simulink library "SCGAnalysis_SignalGenerationLib"  (R2020b)
settings: Solver=VariableStepAuto  StartTime=0.0  StopTime=10.0  RelTol=1e-3
undefined symbols (not defined in the file or in its folder): analyses, fs
settings Model: Creator=Rafael  LastModifiedBy=Rafael

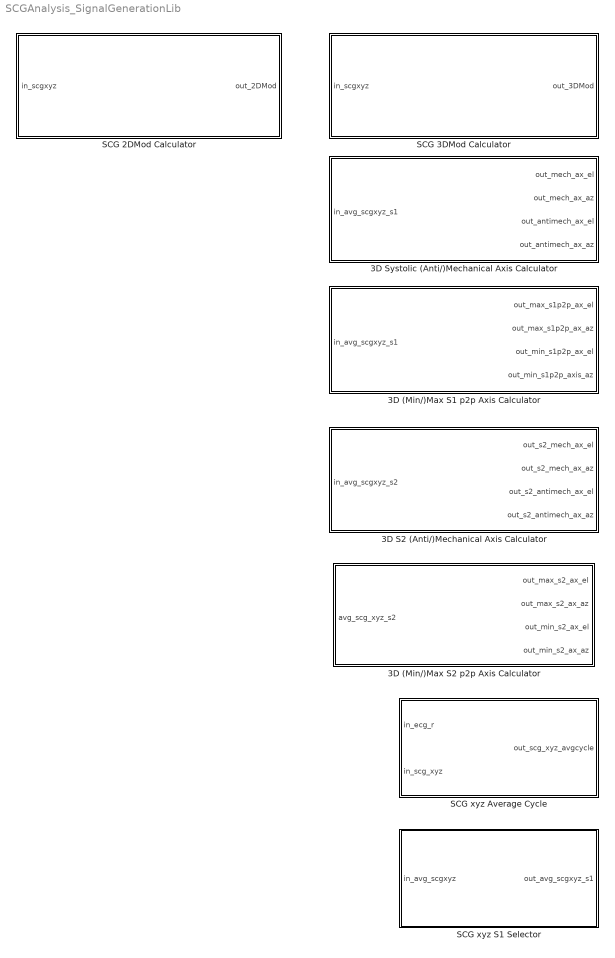
== system SCGAnalysis_SignalGenerationLib ==
  3D (Min/)Max S1 p2p Axis Calculator : Subsystem
      mask Display: image('$imagefile'); % Use "Edit Image" on toolstrip to change.
  3D (Min/)Max S2 p2p Axis Calculator : Subsystem
      mask Display: image('3D Max S2P2P Axis.png'); % Use "Edit Image" on toolstrip to change.
  3D S2 (Anti/)Mechanical Axis Calculator : Subsystem
      mask Display: image('$imagefile'); % Use "Edit Image" on toolstrip to change.
  3D Systolic (Anti/)Mechanical Axis Calculator : Subsystem
      mask Display: image('$imagefile'); % Use "Edit Image" on toolstrip to change.
  SCG 2DMod Calculator : Subsystem  mask{xyz2Dcombo=xz (transverse plane)}
      mask prompts: xyz2Dcombo "2D component combination:"
      mask init:
      | if xyz2Dcombo == 1
      |     param_2Dxyzcombo = 'xy';
      | elseif xyz2Dcombo == 2
      |     param_2Dxyzcombo = 'yz';
      | elseif xyz2Dcombo == 3
      |     param_2Dxyzcombo = 'xz';
      | end
      | 
      | assignin('base','param_2Dxyzcombo', param_2Dxyzcombo)
      mask TypeOptions xyz2Dcombo: xy (coronal plane) | yz (sagittal plane) | xz (transverse plane)
      mask DialogControl DescGroupVar Prompt: 2D Modulus Calculator
      mask DialogControl DescTextVar Prompt: Subsystem to calculate a 2D modulus signal from a user-specified combination of any two of the SCG x, y, or z components.
      mask Display: image('$imagefile'); % Use "Edit Image" on toolstrip to change.
  SCG 3DMod Calculator : Subsystem
      mask Display: image('$imagefile'); % Use "Edit Image" on toolstrip to change.
  SCG xyz Average Cycle : Subsystem
      mask Display: image('$imagefile'); % Use "Edit Image" on toolstrip to change.
  SCG xyz S1 Selector : Subsystem
      mask Display: image('Average S1.png'); % Use "Edit Image" on toolstrip to change.

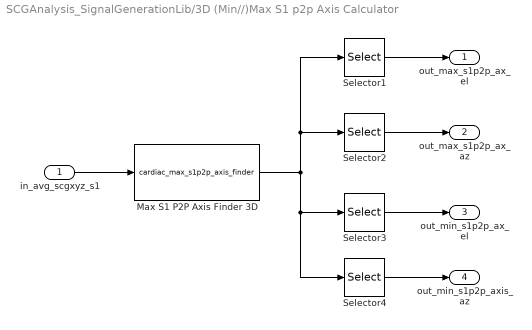
== system SCGAnalysis_SignalGenerationLib/3D (Min//)Max S1 p2p Axis Calculator ==
  in_avg_scgxyz_s1 : Inport
  Max S1 P2P Axis Finder 3D : MATLABFcn  MATLABFcn=cardiac_max_s1p2p_axis_finder  OutputDimensions=4  Output1D=off
  Selector1 : Selector  InputPortWidth=4  IndexOptions=Index vector (dialog)  Indices=[1]  OutputSizes=1
  Selector2 : Selector  InputPortWidth=4  IndexOptions=Index vector (dialog)  Indices=[2]  OutputSizes=1
  Selector3 : Selector  InputPortWidth=4  IndexOptions=Index vector (dialog)  Indices=[3]  OutputSizes=1
  Selector4 : Selector  InputPortWidth=4  IndexOptions=Index vector (dialog)  Indices=[4]  OutputSizes=1
  out_max_s1p2p_ax_el : Outport
  out_max_s1p2p_ax_az : Outport  Port=2
  out_min_s1p2p_ax_el : Outport  Port=3
  out_min_s1p2p_axis_az : Outport  Port=4
  wires:
  in_avg_scgxyz_s1/1 -> Max S1 P2P Axis Finder 3D/1
  Max S1 P2P Axis Finder 3D/1 -> Selector4/1, Selector3/1, Selector1/1, Selector2/1
  Selector1/1 -> out_max_s1p2p_ax_el/1
  Selector2/1 -> out_max_s1p2p_ax_az/1
  Selector4/1 -> out_min_s1p2p_axis_az/1
  Selector3/1 -> out_min_s1p2p_ax_el/1

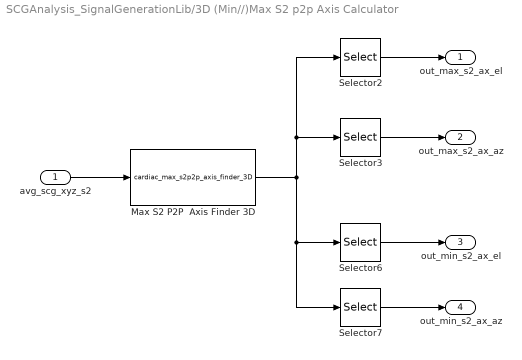
== system SCGAnalysis_SignalGenerationLib/3D (Min//)Max S2 p2p Axis Calculator ==
  avg_scg_xyz_s2 : Inport
  Max S2 P2P  Axis Finder 3D : MATLABFcn  MATLABFcn=cardiac_max_s2p2p_axis_finder_3D  OutputDimensions=4  Output1D=off
  Selector2 : Selector  InputPortWidth=4  IndexOptions=Index vector (dialog)  Indices=[1]  OutputSizes=1
  Selector3 : Selector  InputPortWidth=4  IndexOptions=Index vector (dialog)  Indices=[2]  OutputSizes=1
  Selector6 : Selector  InputPortWidth=4  IndexOptions=Index vector (dialog)  Indices=[3]  OutputSizes=1
  Selector7 : Selector  InputPortWidth=4  IndexOptions=Index vector (dialog)  Indices=[4]  OutputSizes=1
  out_max_s2_ax_el : Outport
  out_max_s2_ax_az : Outport  Port=2
  out_min_s2_ax_el : Outport  Port=3
  out_min_s2_ax_az : Outport  Port=4
  wires:
  avg_scg_xyz_s2/1 -> Max S2 P2P  Axis Finder 3D/1
  Max S2 P2P  Axis Finder 3D/1 -> Selector7/1, Selector6/1, Selector2/1, Selector3/1
  Selector2/1 -> out_max_s2_ax_el/1
  Selector3/1 -> out_max_s2_ax_az/1
  Selector7/1 -> out_min_s2_ax_az/1
  Selector6/1 -> out_min_s2_ax_el/1

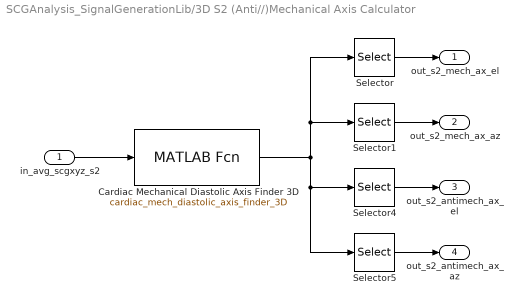
== system SCGAnalysis_SignalGenerationLib/3D S2 (Anti//)Mechanical Axis Calculator ==
  in_avg_scgxyz_s2 : Inport
  Cardiac Mechanical Diastolic Axis Finder 3D : MATLABFcn  MATLABFcn=cardiac_mech_diastolic_axis_finder_3D  OutputDimensions=4  Output1D=off
  Selector : Selector  InputPortWidth=4  IndexOptions=Index vector (dialog)  Indices=[1]  OutputSizes=1
  Selector1 : Selector  InputPortWidth=4  IndexOptions=Index vector (dialog)  Indices=[2]  OutputSizes=1
  Selector4 : Selector  InputPortWidth=4  IndexOptions=Index vector (dialog)  Indices=[3]  OutputSizes=1
  Selector5 : Selector  InputPortWidth=4  IndexOptions=Index vector (dialog)  Indices=[4]  OutputSizes=1
  out_s2_mech_ax_el : Outport
  out_s2_mech_ax_az : Outport  Port=2
  out_s2_antimech_ax_el : Outport  Port=3
  out_s2_antimech_ax_az : Outport  Port=4
  wires:
  in_avg_scgxyz_s2/1 -> Cardiac Mechanical Diastolic Axis Finder 3D/1
  Selector1/1 -> out_s2_mech_ax_az/1
  Selector4/1 -> out_s2_antimech_ax_el/1
  Selector/1 -> out_s2_mech_ax_el/1
  Selector5/1 -> out_s2_antimech_ax_az/1
  Cardiac Mechanical Diastolic Axis Finder 3D/1 -> Selector1/1, Selector/1, Selector4/1, Selector5/1

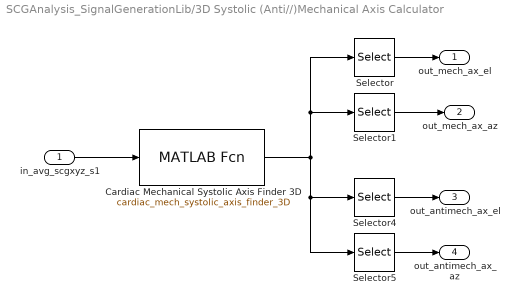
== system SCGAnalysis_SignalGenerationLib/3D Systolic (Anti//)Mechanical Axis Calculator ==
  in_avg_scgxyz_s1 : Inport
  Cardiac Mechanical Systolic Axis Finder 3D : MATLABFcn  MATLABFcn=cardiac_mech_systolic_axis_finder_3D  OutputDimensions=4  Output1D=off
  Selector : Selector  InputPortWidth=4  IndexOptions=Index vector (dialog)  Indices=[1]  OutputSizes=1
  Selector1 : Selector  InputPortWidth=4  IndexOptions=Index vector (dialog)  Indices=[2]  OutputSizes=1
  Selector4 : Selector  InputPortWidth=4  IndexOptions=Index vector (dialog)  Indices=[3]  OutputSizes=1
  Selector5 : Selector  InputPortWidth=4  IndexOptions=Index vector (dialog)  Indices=[4]  OutputSizes=1
  out_mech_ax_el : Outport
  out_mech_ax_az : Outport  Port=2
  out_antimech_ax_el : Outport  Port=3
  out_antimech_ax_az : Outport  Port=4
  wires:
  Cardiac Mechanical Systolic Axis Finder 3D/1 -> Selector5/1, Selector4/1, Selector/1, Selector1/1
  Selector5/1 -> out_antimech_ax_az/1
  Selector/1 -> out_mech_ax_el/1
  Selector4/1 -> out_antimech_ax_el/1
  Selector1/1 -> out_mech_ax_az/1
  in_avg_scgxyz_s1/1 -> Cardiac Mechanical Systolic Axis Finder 3D/1

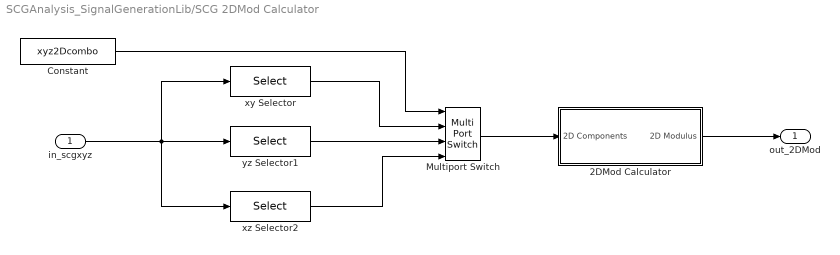
== system SCGAnalysis_SignalGenerationLib/SCG 2DMod Calculator ==
  in_scgxyz : Inport
  2DMod Calculator : Subsystem
  Constant : Constant  Value=xyz2Dcombo
  Multiport Switch : MultiPortSwitch
  xy Selector : Selector  NumberOfDimensions=2  IndexOptions=Select all,Index vector (dialog)  Indices=[1:min(analyses.ecg.RR)],[1 2]  OutputSizes=1,1
  xz Selector2 : Selector  NumberOfDimensions=2  IndexOptions=Select all,Index vector (dialog)  Indices=[1:min(analyses.ecg.RR)],[1 3]  OutputSizes=1,1
  yz Selector1 : Selector  NumberOfDimensions=2  IndexOptions=Select all,Index vector (dialog)  Indices=[1:min(analyses.ecg.RR)],[2 3]  OutputSizes=1,1
  out_2DMod : Outport  VectorParamsAs1DForOutWhenUnconnected=off
  wires:
  2DMod Calculator/1(2D Modulus) -> out_2DMod/1
  in_scgxyz/1 -> xz Selector2/1, xy Selector/1, yz Selector1/1
  Constant/1 -> Multiport Switch/1
  Multiport Switch/1 -> 2DMod Calculator/1(2D Components)
  xy Selector/1 -> Multiport Switch/2
  yz Selector1/1 -> Multiport Switch/3
  xz Selector2/1 -> Multiport Switch/4

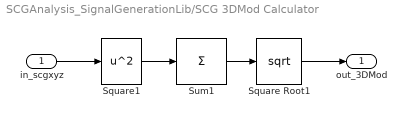
== system SCGAnalysis_SignalGenerationLib/SCG 3DMod Calculator ==
  in_scgxyz : Inport
  Square Root1 : Sqrt  SaturateOnIntegerOverflow=on
  Square1 : Math  Operator=square  SignedPower=on  SaturateOnIntegerOverflow=on
  Sum1 : Sum  Inputs=+  CollapseMode=Specified dimension  CollapseDim=2
  out_3DMod : Outport  VectorParamsAs1DForOutWhenUnconnected=off
  wires:
  Square1/1 -> Sum1/1
  Sum1/1 -> Square Root1/1
  in_scgxyz/1 -> Square1/1
  Square Root1/1 -> out_3DMod/1

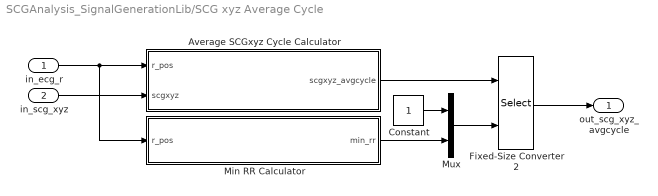
== system SCGAnalysis_SignalGenerationLib/SCG xyz Average Cycle ==
  in_ecg_r : Inport
  in_scg_xyz : Inport  Port=2
  Average SCGxyz Cycle Calculator : MATLAB Function  TreatAsAtomicUnit=on
  Constant : Constant
  Fixed-Size Converter 2 : Selector  NumberOfDimensions=2  IndexOptions=Starting and ending indices (port),Index vector (dialog)  Indices=[1:min(analyses.ecg.RR)],[1 2 3]  OutputSizes=1,1
  Min RR Calculator : MATLAB Function  TreatAsAtomicUnit=on
  Mux : Mux  Inputs=2
  out_scg_xyz_avgcycle : Outport  VectorParamsAs1DForOutWhenUnconnected=off
  wires:
  in_scg_xyz/1 -> Average SCGxyz Cycle Calculator/2(scgxyz)
  in_ecg_r/1 -> Min RR Calculator/1(r_pos), Average SCGxyz Cycle Calculator/1(r_pos)
  Average SCGxyz Cycle Calculator/1(scgxyz_avgcycle) -> Fixed-Size Converter 2/1
  Fixed-Size Converter 2/1 -> out_scg_xyz_avgcycle/1
  Constant/1 -> Mux/1
  Min RR Calculator/1(min_rr) -> Mux/2
  Mux/1 -> Fixed-Size Converter 2/2

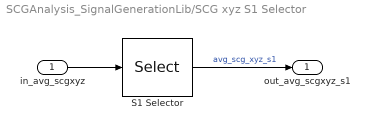
== system SCGAnalysis_SignalGenerationLib/SCG xyz S1 Selector ==
  in_avg_scgxyz : Inport
  S1 Selector : Selector  NumberOfDimensions=2  InputPortWidth=3  IndexOptions=Index vector (dialog),Index vector (dialog)  Indices=[1:fs*0.2],[1 2 3]  OutputSizes=1,1
  out_avg_scgxyz_s1 : Outport
  wires:
  S1 Selector/1 -> out_avg_scgxyz_s1/1  "avg_scg_xyz_s1"
  in_avg_scgxyz/1 -> S1 Selector/1

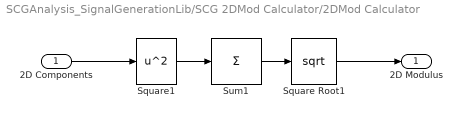
== system SCGAnalysis_SignalGenerationLib/SCG 2DMod Calculator/2DMod Calculator ==
  2D Components : Inport
  Square Root1 : Sqrt  SaturateOnIntegerOverflow=on
  Square1 : Math  Operator=square  SignedPower=on  SaturateOnIntegerOverflow=on
  Sum1 : Sum  Inputs=+  CollapseMode=Specified dimension  CollapseDim=2
  2D Modulus : Outport  VectorParamsAs1DForOutWhenUnconnected=off
  wires:
  Square1/1 -> Sum1/1
  Sum1/1 -> Square Root1/1
  2D Components/1 -> Square1/1
  Square Root1/1 -> 2D Modulus/1

== matlab function SCGAnalysis_SignalGenerationLib/SCG xyz Average Cycle/Average SCGxyz Cycle Calculator ==
  data: r_pos input; scgxyz input; scgxyz_avgcycle output size=[3*fs 3]
function scgxyz_avgcycle  = slk_avg_scgxyz_cycle_calculator(r_pos,scgxyz)
% Simulink function to return the average x,y, and z cycles of the SCG.

% INPUTS:
% r_pos = index positions of the R peaks of the ecg.
% scgxyz = matrix of size [length_scg 3] with the (normally pre-processed) SCG
%          x,y, and z components. The first column corresponds to SCGx, the second
%          to SCGy and the third to SCGz.

% OUTPUT:
% avg_scg_xyz = matrix of size [min_rr 3] with the average SCG cycles of
%               the x,y, and z components. The first column corresponds to SCGx, the second
%               to SCGy and the third to SCGz 


% Calculating number of cycles to be considered in averaging (considered_cycles).
rr_min = min(diff(r_pos)); % Shortest cycle length - all the cycles will but cut down to this length.

if length(scgxyz) > r_pos(end) + rr_min
    considered_cycles = length(r_pos);
else
    considered_cycles = length(r_pos) - 1;
end

scg_x_cycles = zeros(rr_min,considered_cycles);
scg_y_cycles = zeros(rr_min,considered_cycles);
scg_z_cycles = zeros(rr_min,considered_cycles);

fig_scg_average_cycles = figure;

% Isolating and plotting each cycle
for i = 1:considered_cycles
    figure(fig_scg_average_cycles);
    scg_x_cycles(:,i) = scgxyz(r_pos(i):r_pos(i) + rr_min - 1,1);
    scg_y_cycles(:,i) = scgxyz(r_pos(i):r_pos(i) + rr_min - 1,2);
    scg_z_cycles(:,i) = scgxyz(r_pos(i):r_pos(i) + rr_min - 1,3);
    
    % Plotting
    subplot(3,1,1); plot(scg_x_cycles(:,i),'b'); hold on;
    subplot(3,1,2); plot(scg_y_cycles(:,i),'b'); hold on;
    subplot(3,1,3); plot(scg_z_cycles(:,i),'b'); hold on;
end

% Calculating average cycle
avg_scg_x = mean(scg_x_cycles,2);
avg_scg_y = mean(scg_y_cycles,2);
avg_scg_z = mean(scg_z_cycles,2);

% Plotting the average cycle
subplot(3,1,1); plot(avg_scg_x,'k','LineWidth',2); title('Average SCG x'); box off;
subplot(3,1,2); plot(avg_scg_y,'k','LineWidth',2); title('Average SCG y'); ylabel('Amplitude (mg)'); box off;
subplot(3,1,3); plot(avg_scg_z,'k','LineWidth',2); title('Average SCG z'); xlabel('Time (msec)'); box off;

scgxyz_avgcycle = [avg_scg_x avg_scg_y avg_scg_z];
end

== matlab function SCGAnalysis_SignalGenerationLib/SCG xyz Average Cycle/Min RR Calculator ==
  data: r_pos input; min_rr output size=[1]
function min_rr  = slk_min_rr_calculator(r_pos)
% Simulink function to calculate the shortest RR interval from a sequence
% of R peak inputs.

% INPUTS:
% r_pos = index positions of the R peaks of the ecg.

% OUTPUT:
% min_rr = minimum RR interval.

if r_pos % Only enter the function if a valid r_pos sequence is passed to it.
    min_rr = min(diff(r_pos)); % Shortest cycle length - all the cycles will but cut down to this length.
else
    min_rr = 0;
end
end
